simulink model "ESTACAO"  (R2024a)
settings: Solver=VariableStepAuto  StartTime=0.0  StopTime=Inf  RelTol=1e-3
settings Model: Creator=thali  LastModifiedBy=thali

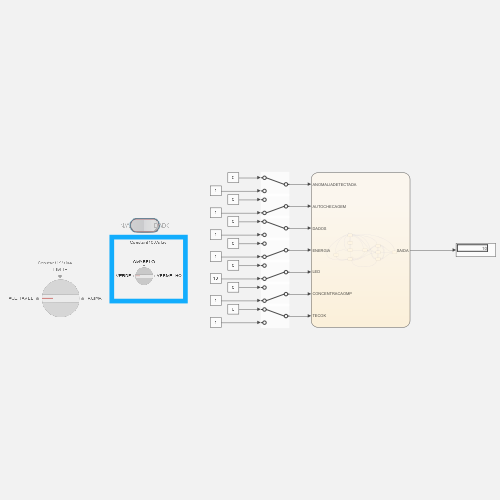
[thumbnail: Simulink's stored preview of the top-level diagram]
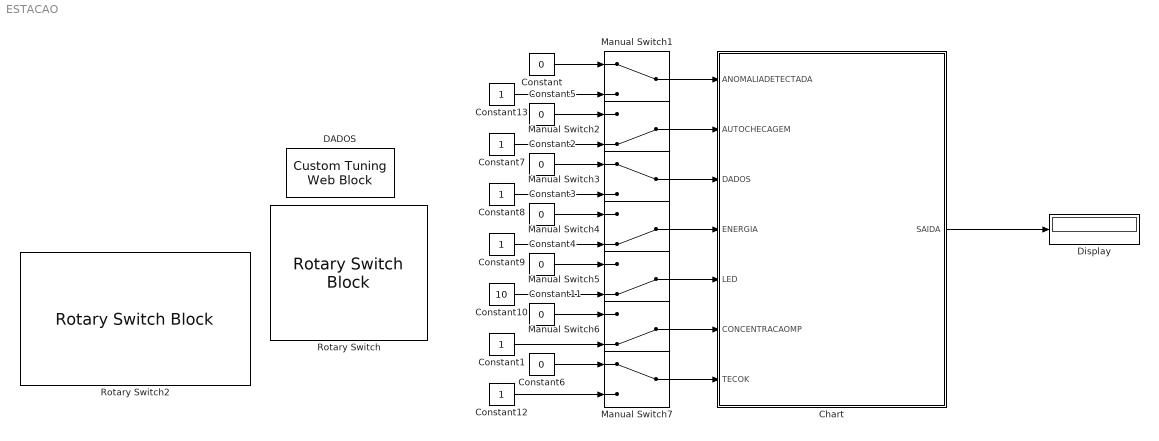
== system ESTACAO ==
  Chart : Stateflow chart  TreatAsAtomicUnit=on
  Constant{,2..6,11} (7 alike) : Constant  Value=0
  Constant{1,7..9,12..13} (6 alike) : Constant
  Constant10 : Constant  Value=10
  DADOS : CustomTuningWebBlock  LabelPosition=Hide  ShowInitialText=on  Configuration="{\"components\":[{\"name\":\"CustomSwitchStateComponent\",\"settings\":{\"position\":[0,0,1,1],\"states\":[{\"HitRegion\":{\"position\":[0,0,0.5,1]},\"Image\":{\"position\":[0.13,0,1,0.75],\"size\":[1,0.75],\"src\":\"data:image\\/svg+xml;base64,PHN2ZyB4bWxucz0iaHR0cDovL3d3dy53My5vcmcvMjAwMC9zdmciIHhtbG5zOnhsaW5rPSJodHRwOi8vd3d3LnczLm9yZy8xOTk5L3hsaW5rIiB2aWV3Qm94PSIwIDAgNzUgMjQuOCI+PGRlZnM+PHN0eWxlPi5jbHMtMXtmaWxsOnVybCgjcmFkaWFsLWdyYWRpZW50KTt9LmNscy0ye2ZpbGw6dXJsKCNyYWRpYWwtZ3JhZGllbnQtMik7fS5jbHMtM3tzdHJva2U6I2IyMDAwMDtzdHJva2Utd2lkdGg6MC4yNXB4O2ZpbGw6dXJsKCNsaW5lYXItZ3JhZGllbnQpO30uY2xzLTR7ZmlsbDp1cmwoI2xpbmVhci1ncmFkaWVudC0yKTt9LmNs ...(+3576 chars)\",\"srcOrientation\":\"Right\"},\"Label\":{\"color\":[0.5019607843137255,0.5019607843137255,0.5019607843137255],\"icon\":{\"size\":[0,0],\"src\":[],\"srcOrientation\":\"Right\"},\"iconPlacement\":\"left\",\"opacity\":1,\"position\":[0.5,0.08],\"show\":true,\"text\":{\"content\":\"N\\/A\",\"font\":\"Helvetica\",\"fontSize\":17.5}},\"Value\":0},{\"HitRegion\":{\"position\":[0,0.5,0.5,1]},\"Image\":{\"position\":[0.13,0,1,0.75],\"size\":[1,0.75],\"src\":\"data:image\\/svg+xml;base64,PHN2ZyB4bWxucz0iaHR0cDovL3d3dy53My5vcmcvMjAwMC9zdmciIHhtbG5zOnhsaW5rPSJodHRwOi8vd3d3LnczLm9yZy8xOTk5L3hsaW5rIiB2aWV3Qm94PSIwIDAgNzUgMjQuOCI+PGRlZnM+PHN0eWxlPi5jbHMtMXtmaWxsOnVybCgjcmFkaWFsLWdyYWRpZW50KTt9LmNscy0ye2ZpbGw6dXJsKCNyYWRpYWwtZ3JhZGllbnQtMik7fS5jbHMtM3tzdHJva2U6I2IyMDAwMDtzdHJva2Utd2lkdGg6MC4yNXB4O2ZpbGw6dXJsKCNsaW5lYXItZ3JhZGllbnQpO30uY2xzLTR7ZmlsbDp1cmwoI2xpbmVhci1ncmFkaWVudC0yKTt9LmNs ...(+3520 chars)\",\"srcOrientation\":\"Right\"},\"Label\":{\"color\":[0.5019607843137255,0.5019607843137255,0.5019607843137255],\"icon\":{\"size\":[0,0],\"src\":[],\"srcOrientation\":\"Right\"},\"iconPlacement\":\"left\",\"opacity\":1,\"position\":[0.5,0.92],\"show\":true,\"text\":{\"content\":\"DADOS\",\"font\":\"Helvetica\",\"fontSize\":17.5}},\"Value\":1}]}},{\"name\":\"BackgroundImageComponent\",\"settings\":{\"image\":{\"size\":[155,70],\"src\":\"default\",\"srcOrientation\":\"Right\"},\"position\":[0,0,1,1],\"scaleMode\":\"0\"}},{\"name\":\"ForegroundImageComponent\",\"settings\":{\"image\":{\"size\":[0,0],\"src\":\"default\",\"srcOrientation\":[]},\"isForeground\":1,\"position\":[0,0,1,1],\"scaleMode\":\"0\"}}],\"settings\":{\"BindingType\":\"param\",\"backgroundColor\":[0,0,255,\"1\"],\"backgroundOffset\":0.14,\"fixedAspectRatio\":\"on\",\"foregroundColor\":[234,234,234],\"showBackgroundColor\":false,\"variant\":\"rocker\",\"version\":\"R2023a\"},\"type\":\"Switch\"}"
  Display : Display
  Manual Switch1 : ManualSwitch
  Manual Switch{2,4..6} (4 alike) : ManualSwitch  CurrentSetting=0
  Manual Switch3 : ManualSwitch
  Manual Switch7 : ManualSwitch
  Rotary Switch : RotarySwitchBlock
      settings: Values={{'VERDE', 'AMARELO', 'VERMELHO'}, [10 20 30]}
  Rotary Switch2 : RotarySwitchBlock
      settings: Values={{'ACEITAVEL', 'LIMITE', 'ACIMA'}, [1 2 3]}
  wires:
  Chart/1(SAIDA) -> Display/1
  Manual Switch1/1 -> Chart/1(ANOMALIADETECTADA)
  Manual Switch2/1 -> Chart/2(AUTOCHECAGEM)
  Manual Switch3/1 -> Chart/3(DADOS)
  Manual Switch4/1 -> Chart/4(ENERGIA)
  Manual Switch5/1 -> Chart/5(LED)
  Manual Switch7/1 -> Chart/7(TECOK)
  Constant/1 -> Manual Switch1/1
  Constant13/1 -> Manual Switch1/2
  Constant2/1 -> Manual Switch3/1
  Constant3/1 -> Manual Switch4/1
  Constant4/1 -> Manual Switch5/1
  Constant6/1 -> Manual Switch7/1
  Constant7/1 -> Manual Switch2/2
  Constant8/1 -> Manual Switch3/2
  Constant9/1 -> Manual Switch4/2
  Constant10/1 -> Manual Switch5/2
  Constant12/1 -> Manual Switch7/2
  Constant5/1 -> Manual Switch2/1
  Manual Switch6/1 -> Chart/6(CONCENTRACAOMP)
  Constant11/1 -> Manual Switch6/1
  Constant1/1 -> Manual Switch6/2

== stateflow chart ESTACAO/Chart ==
  state DESENERGIZADO
  state DESLIGADO
  state LEDVERDE
  state AUTOCHECAGEM
  state LEITURA
  state LED1AMARELO
  state COLETA
    DADOS
  state REINICIAR
  state LED2VERMELHO
  state ALERTA
  (default) -> DESENERGIZADO
  COLETA -> DESENERGIZADO : [ENERGIA == 0]{SAIDA = 0}
  ALERTA -> DESENERGIZADO [order 3] : [ENERGIA == 0]{SAIDA = 0}
  LED2VERMELHO -> DESENERGIZADO [order 4] : [ENERGIA == 0]{SAIDA = 0}
  REINICIAR -> DESENERGIZADO [order 2] : [ENERGIA == 0]{SAIDA = 0}
  LED1AMARELO -> DESENERGIZADO [order 4] : [ENERGIA == 0]{SAIDA = 0}
  LEDVERDE -> DESENERGIZADO [order 4] : [ENERGIA == 0]{SAIDA = 0}
  AUTOCHECAGEM -> DESENERGIZADO [order 4] : [ENERGIA == 0]{SAIDA = 0}
  LEITURA -> DESENERGIZADO [order 5] : [ENERGIA == 0]{SAIDA = 0}
  DESENERGIZADO -> DESLIGADO : [ENERGIA == 1]{SAIDA = 0}
  DESLIGADO -> DESENERGIZADO [order 1] : [ENERGIA == 0]{SAIDA = 0}
  DESLIGADO -> AUTOCHECAGEM [order 2] : [ENERGIA == 1 && AUTOCHECAGEM == 1]{SAIDA = 0}
  AUTOCHECAGEM -> DESLIGADO [order 1] : [ENERGIA == 0]{SAIDA = 0}
  LED2VERMELHO -> LEDVERDE [order 2] : [ENERGIA == 1 && CONCENTRACAOMP == 1]{SAIDA = 10}
  LEITURA -> LEDVERDE [order 1] : [ENERGIA == 1 && CONCENTRACAOMP == 1]{SAIDA = 10}
  LEDVERDE -> COLETA [order 5] : [ENERGIA == 1 && DADOS == 1]{SAIDA = 100}
  LEDVERDE -> LED2VERMELHO [order 2] : [ENERGIA == 1 && CONCENTRACAOMP == 3]{SAIDA = 30}
  LEDVERDE -> ALERTA [order 3] : [ENERGIA == 1 && ANOMALIADETECTADA == 1]{SAIDA = 2}
  LEDVERDE -> LED1AMARELO [order 1] : [ENERGIA == 1 && CONCENTRACAOMP == 2]{SAIDA = 20}
  LED1AMARELO -> LEDVERDE [order 1] : [ENERGIA == 1 && CONCENTRACAOMP == 1]{SAIDA = 10}
  REINICIAR -> AUTOCHECAGEM [order 1] : [ENERGIA == 1 && AUTOCHECAGEM == 1]{SAIDA = 0}
  AUTOCHECAGEM -> LEITURA [order 2] : [ENERGIA == 1 && ANOMALIADETECTADA == 0]{SAIDA = 1}
  LEITURA -> LED1AMARELO [order 2] : [ENERGIA == 1 && CONCENTRACAOMP == 2]{SAIDA = 20}
  LEITURA -> LED2VERMELHO [order 3] : [ENERGIA == 1 && CONCENTRACAOMP == 3]{SAIDA = 30}
  AUTOCHECAGEM -> ALERTA [order 3] : [ENERGIA == 1 && ANOMALIADETECTADA == 1]{SAIDA = 2}
  LEITURA -> ALERTA [order 4] : [ENERGIA == 1 && ANOMALIADETECTADA == 1]{SAIDA = 2}
  LED1AMARELO -> COLETA [order 5] : [ENERGIA == 1 && DADOS == 1]{SAIDA = 100}
  LED1AMARELO -> ALERTA [order 3] : [ENERGIA == 1 && ANOMALIADETECTADA == 1]{SAIDA = 2}
  LED2VERMELHO -> COLETA [order 5] : [ENERGIA == 1 && DADOS == 1]{SAIDA = 100}
  LED1AMARELO -> LED2VERMELHO [order 2] : [ENERGIA == 1 && CONCENTRACAOMP == 3]{SAIDA = 30}
  LED2VERMELHO -> LED1AMARELO [order 1] : [ENERGIA == 1 && CONCENTRACAOMP == 2]{SAIDA = 20}
  ALERTA -> REINICIAR [order 2] : [ENERGIA == 1 && ANOMALIADETECTADA == 0 && TECOK == 1]{SAIDA = 3}
  ALERTA -> ALERTA [order 1] : [ENERGIA == 1 && ANOMALIADETECTADA == 1 && TECOK == 0]{SAIDA = 2}
  LED2VERMELHO -> ALERTA [order 3] : [ENERGIA == 1 && ANOMALIADETECTADA == 1]{SAIDA = 2}
  data: SAIDA output; ANOMALIADETECTADA input; AUTOCHECAGEM input; DADOS input; ENERGIA input; LED input; CONCENTRACAOMP input; TECOK input
